simulink model "peak_current_mode_1phase"  (R2021b)
settings: Solver=VariableStepAuto  StartTime=0.0  StopTime=10  RelTol=1e-3
libraries: spsVoltageMeasurementLib x2, spsACVoltageSourceLib x1, spsCurrentMeasurementLib x1, spsDCMachineLib x1, spsDCVoltageSourceLib x1, spsUniversalBridgeLib x1, spspowerguiLib x1
settings Model: NumberOfSteps=1000  Creator=Göktuğ  LastModifiedBy=Göktuğ

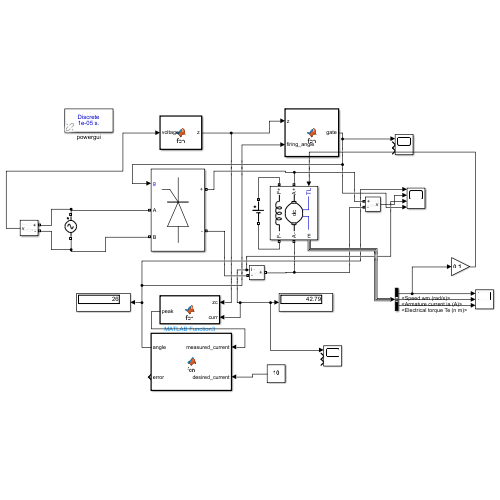
[thumbnail: Simulink's stored preview of the top-level diagram]
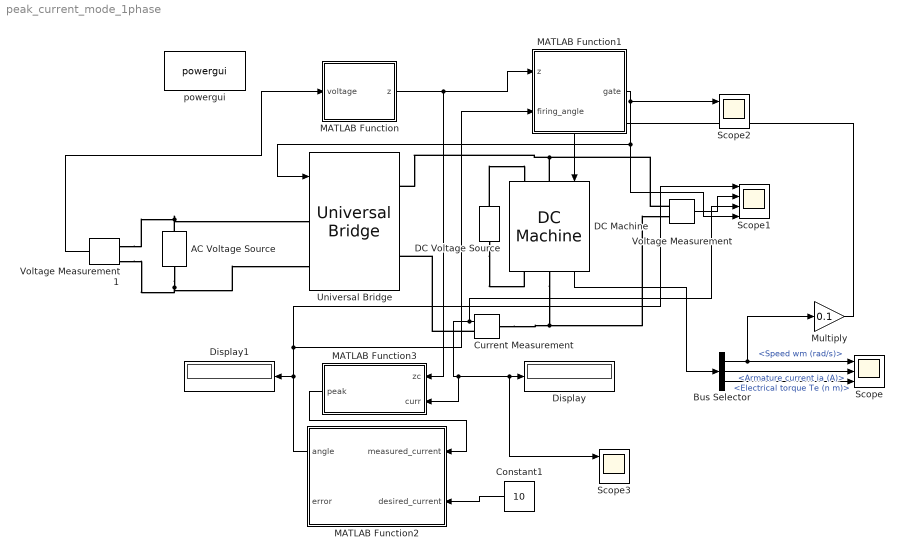
== system peak_current_mode_1phase ==
  AC Voltage Source : spsACVoltageSourceLib/AC Voltage Source  Amplitude=230  Phase=0  Frequency=50  SampleTime=0  Measurements=None  BusType=swing  Pref=10e3  Qref=0  Qmin=-inf  Qmax=+inf
  Bus Selector : BusSelector  OutputSignals=Speed wm (rad/s),Armature current ia (A),Electrical torque Te (n m)
  Constant1 : Constant  Value=10
  Current Measurement : spsCurrentMeasurementLib/Current Measurement  PhasorSimulation=off  OutputType=Complex  PSBequivalent=0
  DC Machine : spsDCMachineLib/DC Machine  PresetModel=No  MechanicalLoad=Torque TL  FieldType=Wound  ShowDetailedParameters=on  MeasurementBus=off  RLa="[ 0.8  12.5e-3]"  RLf="[ 240  120]"  Laf=1.8  MachineConstant=Torque constant (N.m/A)  Ke=1.8  Kt=1.8  J=1  Bm=0  Tf=0  w0=0  Ifinit=0.625  TsPowergui=0  TsBlock=-1
  DC Voltage Source : spsDCVoltageSourceLib/DC Voltage Source  Amplitude=150  Measurements=None
  Display : Display
  Display1 : Display
  MATLAB Function : MATLAB Function  TreatAsAtomicUnit=on
  MATLAB Function1 : MATLAB Function  TreatAsAtomicUnit=on
  MATLAB Function2 : MATLAB Function  TreatAsAtomicUnit=on
  MATLAB Function3 : MATLAB Function  TreatAsAtomicUnit=on
  Multiply : Gain  Gain=0.1
  Scope : Scope  NumInputPorts=3
  Scope1 : Scope  NumInputPorts=4
  Scope2 : Scope  NumInputPorts=3
  Scope3 : Scope  NumInputPorts=3
  Universal Bridge : spsUniversalBridgeLib/Universal Bridge  Arms=2  SnubberResistance=1e5  SnubberCapacitance=inf  Device=Thyristors  Ron=1e-3  Lon=0  ForwardVoltages="[  0  0  ]"  ForwardVoltage=0  GTOparameters=[ 10e-6 , 20e-6 ]  IGBTparameters=[ 1e-6 , 2e-6 ]  Measurements=None  Measurements_2=None  converterType=Rectifier
  Voltage Measurement : spsVoltageMeasurementLib/Voltage Measurement  PhasorSimulation=off  OutputType=Complex  PSBequivalent=0
  Voltage Measurement1 : spsVoltageMeasurementLib/Voltage Measurement  PhasorSimulation=off  OutputType=Complex  PSBequivalent=0
  powergui : spspowerguiLib/powergui  Priority=1  SimulationMode=Discrete  SampleTime=10e-6  frequency=60  Iterations=50  frequencyindice=0  Pbase=100e6  ErrMax=1e-4  UnitsV=kV  UnitsW=MW  buscounter=0  FunctionMessages=off  echomessages=off  EnableUseOfTLC=off  CurrentSourceSwitches=off  DisableSnubberDevices=off  DisableRonSwitches=off  DisableVfSwitches=off  DisplayEquations=off  AutomaticDiscreteSolvers=off  SolverType=Tustin/Backward Euler (TBE)  Interpol=off  ExternalGateDelay=off  methode=off  Ts=100  x0status=blocks  SPID=on  SwTol=0  HookPort=off  NonlinearTolerance=1e-4  nMaxIteration=100  ContinueOnMaxIteration=off  RestoreLinks=warning  ResistiveCurrentMeasurement=off  Frange=[0:2:500]  Ylog=off  Xlog=on  ShowGrid=off  save=off  variable=ZData  structure=0  ZoomFFT=off  StartTime=0.0  cycles=1  DisplayStyle=1  fundamental=60  FreqAxis=off  MaxFrequency=1000  frequencyindicesteady=1  RmsSteady=1  display=off
  wires:
  MATLAB Function/1(z) -> MATLAB Function3/1(zc), MATLAB Function1/1(z)
  MATLAB Function1/1(gate) -> Scope1/4, Universal Bridge/1, Scope2/1
  Voltage Measurement/1 -> Scope1/2
  Current Measurement/1 -> Scope1/3, MATLAB Function3/2(curr), Scope3/1, Display/1
  Constant1/1 -> MATLAB Function2/2(desired_current)
  DC Machine/1 -> Bus Selector/1
  Bus Selector/1 -> Multiply/1, Scope/1  "<Speed wm (rad/s)>"
  Bus Selector/2 -> Scope/2  "<Armature current ia (A)>"
  Bus Selector/3 -> Scope/3  "<Electrical torque Te (n m)>"
  Multiply/1 -> DC Machine/1
  Voltage Measurement1/1 -> MATLAB Function/1(voltage)
  MATLAB Function2/1(angle) -> MATLAB Function1/2(firing_angle), Scope1/1, Display1/1
  MATLAB Function3/1(peak) -> MATLAB Function2/1(measured_current)
  connections:
  DC Voltage Source/RConn1 -- DC Machine/LConn2
  DC Voltage Source/LConn1 -- DC Machine/RConn2
  Voltage Measurement/LConn1 -- DC Machine/LConn1 -- Universal Bridge/RConn1
  Current Measurement/LConn1 -- Voltage Measurement/LConn2 -- DC Machine/RConn1
  Current Measurement/RConn1 -- Universal Bridge/RConn2
  AC Voltage Source/RConn1 -- Voltage Measurement1/LConn1 -- Universal Bridge/LConn1
  AC Voltage Source/LConn1 -- Voltage Measurement1/LConn2 -- Universal Bridge/LConn2

== matlab function peak_current_mode_1phase/MATLAB Function1 ==
  data: z input; gate output size=[1 4]; firing_angle input
function gate = fcn(z, firing_angle)

persistent angle_pA;

if isempty(angle_pA)
    angle_pA = 0;
end

d2r=pi/180;
r2d=180/pi;


if z==1 %sync first phase
    angle_pA = 0;
else
    angle_pA = angle_pA + 0.18;
end

%bridge config is 1 3 
%                 2 4

if(firing_angle<179 && r2d*angdiff((firing_angle)*d2r,angle_pA*d2r)>0 && r2d*angdiff((firing_angle+180)*d2r,angle_pA*d2r)<0)%step1  
    gate_sig = [1 0 0 1];
elseif(firing_angle<179 && r2d*angdiff((firing_angle+180)*d2r,angle_pA*d2r)>0 && r2d*angdiff((firing_angle+360)*d2r,angle_pA*d2r)<0)%step2    
    gate_sig = [0 1 1 0];
else
    gate_sig = [0 0 0 0];
end



gate = gate_sig;


end

== matlab function peak_current_mode_1phase/MATLAB Function ==
  data: voltage input; z output
function z   = fcn( voltage)
    
    persistent past_voltage;
    
    if isempty(past_voltage)
        past_voltage = 0;
    end

    if(past_voltage < 0 && voltage>=0)
        z=1;
    else
        z=0;
    end
    past_voltage = voltage;
end

== matlab function peak_current_mode_1phase/MATLAB Function2 ==
  data: measured_current input; desired_current input; angle output; error output
function [angle, error]= fcn(measured_current,desired_current)
persistent firing_angle;
persistent old_current;

if(isempty(firing_angle))
    firing_angle = 180;
end
if(isempty(old_current))
    old_current = 0;
end

%lets make a cheat, we know that our sample time, 10uS, for one step we need 20mS/6 time which is 3.33mS and app 333step call for our function
%why we are making cheat? because i dont know how to sync the
%measurements, in current configration we are makking measurements in
%random times. This means that we have to somehow, calculate it mean value
%or rms value. Making it causes unnecessary computation, lets assume that
%inductor current is triangular wave and take the middle point as 167.
%measurement. Then by using only every 167. measurement we can calculate
%the current, but this causes a problem. Depending on the firing angle
%actually this number should move. (In a mcu it is just a timer trick but
%in matlab it is really complicated for me) So my last decision is adding
%an adc trigger input, i will create the trigger using firing angle block
%and when it is 1 i will calculate the next firing angle.
if( old_current~=measured_current || firing_angle == 180)
    old_current = measured_current;
    if(desired_current>measured_current)
        firing_angle = firing_angle - 2;
    elseif(measured_current>desired_current)
        firing_angle = firing_angle + 2;
    end
    if(firing_angle<0)
        firing_angle = 0;
    elseif(firing_angle>180)
        firing_angle=180;
    end
end
    error = desired_current - measured_current;
    angle = firing_angle;
end

== matlab function peak_current_mode_1phase/MATLAB Function3 ==
  data: zc input; curr input; peak output
function peak = fcn(zc,curr)
persistent current;
persistent out;
if(isempty(current))
    current = 0;
end
if(isempty(out))
    out = 0;
end
if(curr>current)
    current = curr;
end

if(zc==1)
    out = current;
    current = 0;
end
peak = out;
end
